simulink model "miniProject1"  (Simulink 7.7)
settings: Solver=ode45  StartTime=0.0  StopTime=10.0  RelTol=1e-3
libraries: simulink x1
settings Model: Creator=jiannianweng  LastModifiedBy=jiannianweng

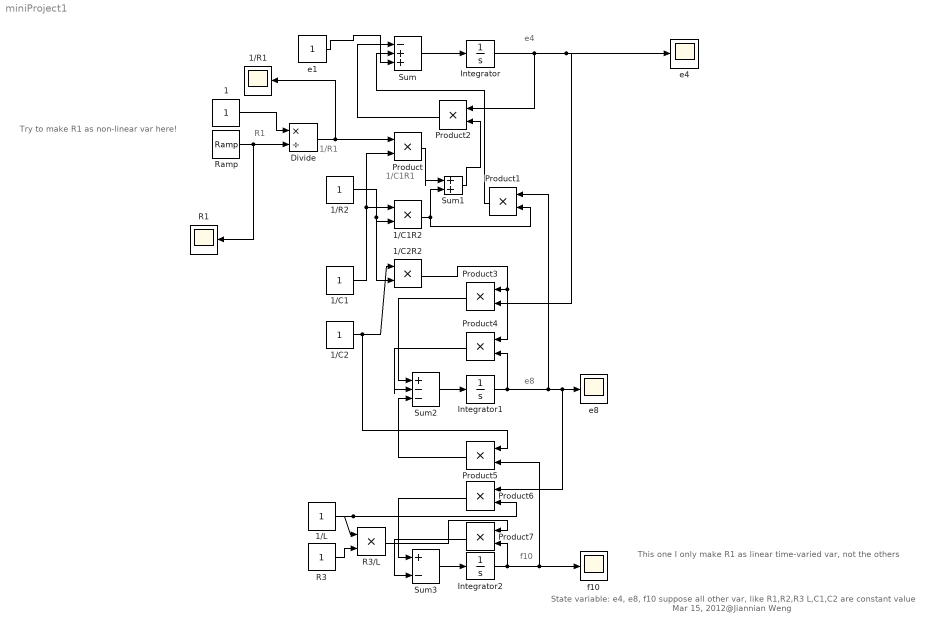
== system miniProject1 ==
  note: e4
  note: e8
  note: f10
  note: 1/C1R1
  note: State variable: e4, e8, f10
      | suppose all other var, like R1,R2,R3
      | L,C1,C2 are constant value
      | Mar 15, 2012@Jiannian Weng
  note: Try to make R1 as non-linear var here!
  note: R1
  note: 1/R1
  note: This one I only make R1 as linear time-varied var, not the others
  1 : Constant
  1/C1 : Constant
  1/C1R2 : Product  RndMeth=Zero
  1/C2 : Constant
  1/C2R2 : Product  RndMeth=Zero
  1/L : Constant
  1/R1 : Scope
      settings: SaveName=ScopeData3
  1/R2 : Constant
  Divide : Product  Inputs=*/
  Integrator : Integrator
  Integrator1 : Integrator
  Integrator2 : Integrator
  Product{,1..7} (8 alike) : Product  RndMeth=Zero
  R1 : Scope
      settings: SaveName=ScopeData4
  R3 : Constant
  R3/L : Product  RndMeth=Zero
  Ramp : simulink/Sources/Ramp  SystemSampleTime=-1  slope=1  start=0  X0=1
  Sum : Sum  Inputs=|-++
  Sum1 : Sum  Inputs=|++
  Sum2 : Sum  Inputs=|+--
  Sum3 : Sum  Inputs=|+-
  e1 : Constant
  e4 : Scope
  e8 : Scope
  f10 : Scope
      settings: SaveName=ScopeData2
  wires:
  Integrator/1 -> Product2/1, e4/1, Product3/2
  Integrator1/1 -> Product1/1, e8/1, Product6/1, Product4/2
  Integrator2/1 -> f10/1, Product5/2, Product7/2
  Sum/1 -> Integrator/1
  e1/1 -> Sum/3
  1/C1/1 -> Product/2, 1/C1R2/1
  1/R2/1 -> 1/C1R2/2, 1/C2R2/2
  Product/1 -> Sum1/1
  1/C1R2/1 -> Sum1/2, Product1/2
  Sum1/1 -> Product2/2
  Product2/1 -> Sum/1
  Product1/1 -> Sum/2
  1/C2/1 -> 1/C2R2/1, Product5/1
  1/C2R2/1 -> Product3/1, Product4/1
  Sum2/1 -> Integrator1/1
  Product3/1 -> Sum2/1
  Product4/1 -> Sum2/2
  Product5/1 -> Sum2/3
  Sum3/1 -> Integrator2/1
  1/L/1 -> Product6/2, R3/L/1
  Product6/1 -> Sum3/1
  R3/1 -> R3/L/2
  R3/L/1 -> Product7/1
  Product7/1 -> Sum3/2
  Divide/1 -> Product/1, 1/R1/1
  1/1 -> Divide/1
  Ramp/1 -> Divide/2, R1/1
